simulink model "psk_model_coded"  (R2023a)
settings: Solver=FixedStepDiscrete  StartTime=0.0  StopTime=1e5  FixedStep=1  RelTol=1e-3
values from neighbouring files (symbols this model uses):
  M = M_values(mod_idx)    [run_ber_sweep.m]
undefined symbols (not defined in the file or in its folder): dvbs2ldpc, Ts
libraries: commsink2 x2, simulink x2, commblkcod2 x2, commcnvcod2 x2, commdigbbndpm3 x2, commchan3 x1, commrandsrc3 x1
settings Model: Creator=aleks  LastModifiedBy=aleks

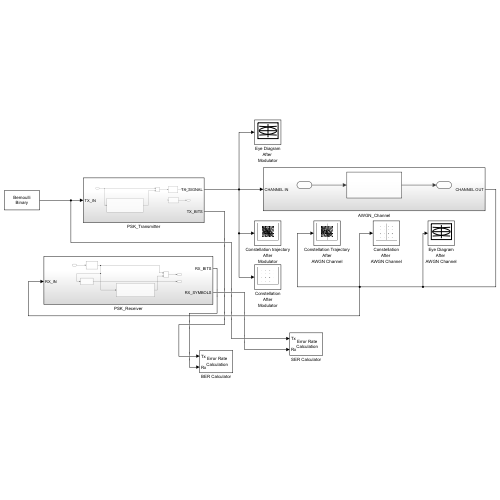
[thumbnail: Simulink's stored preview of the top-level diagram]
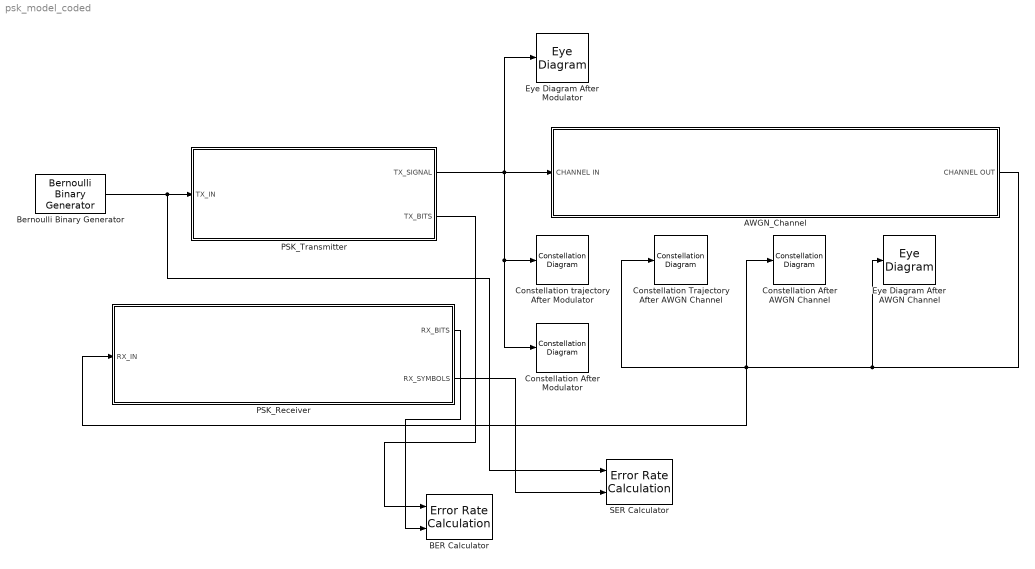
== system psk_model_coded ==
  AWGN_Channel : Subsystem
  BER Calculator : commsink2/Error Rate Calculation  N=0  st_delay=0  cp_mode=Entire frame  subframe=[]  PMode=Workspace  WsName=ber_out  RsMode2=off  stop=off  numErr=100  maxBits=1e6
  Bernoulli Binary Generator : commrandsrc3/Bernoulli Binary Generator  ProbabilityOfZero=bern_prob  SeedSource=Auto  Seed=0  SampleTime=Ts  SamplesPerFrame=1  OutputDataType=double  SimulateUsing=Interpreted execution
  Constellation After Modulator : ConstellationDiagram  WindowPosition=[2.000000,50.000000,766.000000,881.000000,]  Visible=on  ScopeFrameLocation=window  SymbolsToDisplaySource=Property  SymbolsToDisplay=1000  XLimits=[-1.46,1.46]  YLimits=[-1.38,1.38]  ShowReferenceConstellation=off
  Constellation After AWGN Channel : ConstellationDiagram  WindowPosition=[770.000000,50.000000,766.000000,881.000000,]  Visible=on  ScopeFrameLocation=window  SymbolsToDisplaySource=Property  SymbolsToDisplay=1000  XLimits=[-1.46,1.46]  YLimits=[-1.38,1.38]  ShowReferenceConstellation=off
  Constellation Trajectory After AWGN Channel : ConstellationDiagram  WindowPosition=[770.000000,50.000000,766.000000,881.000000,]  Visible=on  ScopeFrameLocation=window  SymbolsToDisplaySource=Property  SymbolsToDisplay=1000  ReferenceConstellation=QPSK  XLimits=[-1.46,1.46]  YLimits=[-1.38,1.38]  ShowTrajectory=on  ShowReferenceConstellation=off
  Constellation trajectory After Modulator : ConstellationDiagram  WindowPosition=[2.000000,50.000000,766.000000,881.000000,]  Visible=on  ScopeFrameLocation=window  SymbolsToDisplaySource=Property  SymbolsToDisplay=1000  ReferenceConstellation=QPSK  XLimits=[-1.46,1.46]  YLimits=[-1.38,1.38]  ShowTrajectory=on  ShowReferenceConstellation=off
  Eye Diagram After AWGN Channel : EyeDiagram
  Eye Diagram After Modulator : EyeDiagram
  PSK_Receiver : Subsystem
  PSK_Transmitter : Subsystem
  SER Calculator : commsink2/Error Rate Calculation  N=0  st_delay=0  cp_mode=Entire frame  subframe=[]  PMode=Workspace  WsName=ser_out  RsMode2=off  stop=off  numErr=100  maxBits=1e6
  wires:
  PSK_Transmitter/1(TX_SIGNAL) -> Constellation After Modulator/1, Constellation trajectory After Modulator/1, Eye Diagram After Modulator/1, AWGN_Channel/1(CHANNEL IN)
  AWGN_Channel/1(CHANNEL OUT) -> Eye Diagram After AWGN Channel/1, PSK_Receiver/1(RX_IN), Constellation After AWGN Channel/1, Constellation Trajectory After AWGN Channel/1
  Bernoulli Binary Generator/1 -> SER Calculator/1, PSK_Transmitter/1(TX_IN)
  PSK_Receiver/1(RX_BITS) -> BER Calculator/2
  PSK_Transmitter/2(TX_BITS) -> BER Calculator/1
  PSK_Receiver/2(RX_SYMBOLS) -> SER Calculator/2

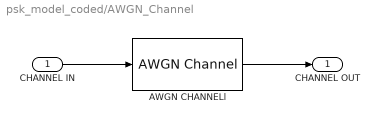
== system psk_model_coded/AWGN_Channel ==
  CHANNEL IN : Inport
  AWGN CHANNELl : commchan3/AWGN Channel  LegacyMode=off  NoiseMethod="Signal to noise ratio  (Eb/No)"  noiseMode="Signal to noise ratio  (SNR)"  EbNo=EbNo_curr  EsNo=10  SNR=10  BitsPerSymbol=log2(M)  SignalPower=1  SamplesPerSymbol=1  SymbolPeriod=1  VarianceSource=Parameter  Variance=1  RandomStream=Global stream  Seed=67  SimulateUsing=Code generation
  CHANNEL OUT : Outport
  wires:
  CHANNEL IN/1 -> AWGN CHANNELl/1
  AWGN CHANNELl/1 -> CHANNEL OUT/1

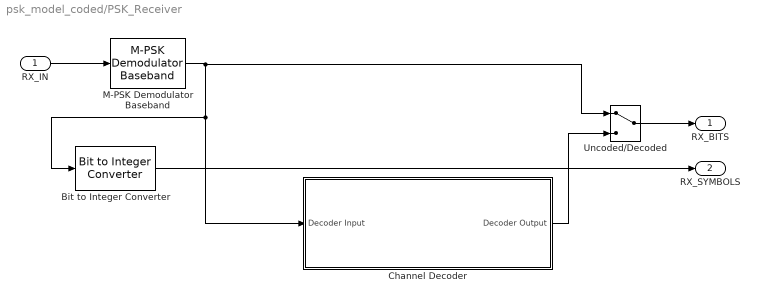
== system psk_model_coded/PSK_Receiver ==
  RX_IN : Inport
  Bit to Integer Converter : simulink/Logic and Bit Operations/Bit to Integer Converter  nbits=log2(M)  bitOrder=MSB first  signedOutputValues=Unsigned  outDtype=Inherit via internal rule  outDtypeSigned=Inherit via internal rule
  Channel Decoder : Subsystem
  M-PSK Demodulator Baseband : commdigbbndpm3/M-PSK Demodulator Baseband  M=M  OutType=Bit  DecType=Hard decision  VarSource=Dialog  Variance=1  Dec=Gray  Mapping=[0:7]  Ph=phase_offset  outDtype1=Inherit via internal rule  outDtype2=Inherit via internal rule  derotateFactorWordLen=16  derotateFactorDataTypeStr=Inherit: Same word length as input  derotateFactorLastDataTypeStr=Inherit: Same word length as input
  Uncoded/Decoded : ManualSwitch
  RX_BITS : Outport
  RX_SYMBOLS : Outport  Port=2
  wires:
  RX_IN/1 -> M-PSK Demodulator Baseband/1
  Bit to Integer Converter/1 -> RX_SYMBOLS/1
  M-PSK Demodulator Baseband/1 -> Uncoded/Decoded/1, Channel Decoder/1(Decoder Input), Bit to Integer Converter/1
  Channel Decoder/1(Decoder Output) -> Uncoded/Decoded/2
  Uncoded/Decoded/1 -> RX_BITS/1

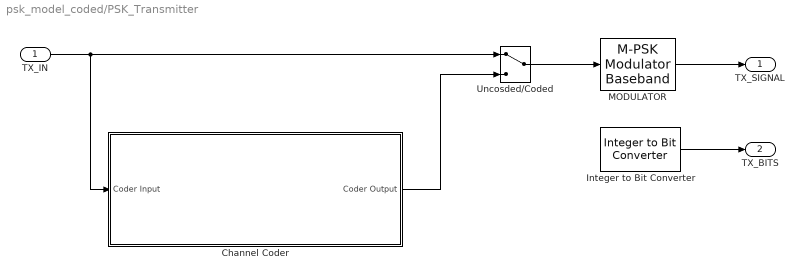
== system psk_model_coded/PSK_Transmitter ==
  TX_IN : Inport
  Channel Coder : Subsystem
  Integer to Bit Converter : simulink/Logic and Bit Operations/Integer to Bit Converter  nbits=log2(M)  signedInputValues=Unsigned  bitOrder=MSB first  outDtype=Inherit via internal rule
  MODULATOR : commdigbbndpm3/M-PSK Modulator Baseband  M=M  InType=Integer  Enc=Gray  Mapping=[0:7]  Ph=phase_offset  outDtype=double  outWordLen=16  outUDDataType=sfix(16)  outFracLenMode=Best precision  outFracLen=15  outDataTypeStr=double  outLastDataTypeStr=double
  Uncosded/Coded : ManualSwitch
  TX_SIGNAL : Outport
  TX_BITS : Outport  Port=2
  wires:
  MODULATOR/1 -> TX_SIGNAL/1
  Integer to Bit Converter/1 -> TX_BITS/1
  TX_IN/1 -> Channel Coder/1(Coder Input), Uncosded/Coded/1
  Channel Coder/1(Coder Output) -> Uncosded/Coded/2
  Uncosded/Coded/1 -> MODULATOR/1

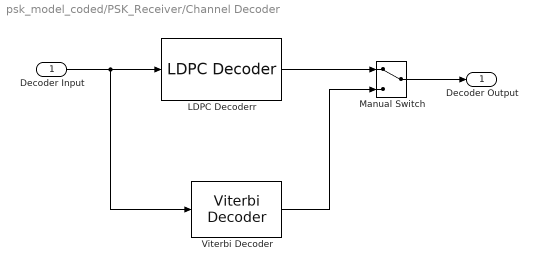
== system psk_model_coded/PSK_Receiver/Channel Decoder ==
  Decoder Input : Inport
  LDPC Decoderr : commblkcod2/LDPC Decoder  ParityCheckMat=dvbs2ldpc(1/2)  OutputFmt=Information part  DecisionType=Hard decision  OutputDataType=double  NumIter=50  DoParityCheck=off  OutputNumIter=off  OutputFinalChecks=off
  Manual Switch : ManualSwitch
  Viterbi Decoder : commcnvcod2/Viterbi Decoder  trellis=poly2trellis(7, [171 133])  isPunctured=off  punctureVector=[1; 1; 0; 1; 0; 1]  erasures=off  dectype=Hard decision  nsdecb=4  runSigValErrCheck=off  tbdepth=34  opmode=Continuous  reset=off  delayedResetAction=off  smWordLength=16  outDataType=Inherit via internal rule
  Decoder Output : Outport
  wires:
  Decoder Input/1 -> Viterbi Decoder/1, LDPC Decoderr/1
  LDPC Decoderr/1 -> Manual Switch/1
  Viterbi Decoder/1 -> Manual Switch/2
  Manual Switch/1 -> Decoder Output/1

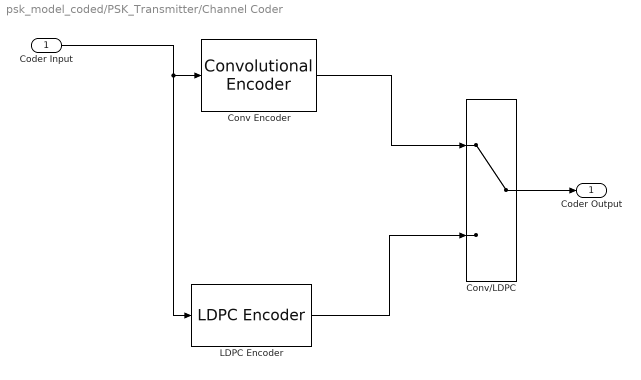
== system psk_model_coded/PSK_Transmitter/Channel Coder ==
  Coder Input : Inport
  Conv Encoder : commcnvcod2/Convolutional Encoder  trellis=poly2trellis(7, [171 133])  opMode=Continuous  DelayedResetAction=off  hasIniStPort=off  hasFinStPort=off  usePuncVector=off  punctureVector=[1; 1; 0; 1; 0; 1]  reset=Unused parameter value
  Conv/LDPC : ManualSwitch
  LDPC Encoder : commblkcod2/LDPC Encoder  ParityCheckMat=dvbs2ldpc(1/2)
  Coder Output : Outport
  wires:
  Conv Encoder/1 -> Conv/LDPC/1
  LDPC Encoder/1 -> Conv/LDPC/2
  Coder Input/1 -> LDPC Encoder/1, Conv Encoder/1
  Conv/LDPC/1 -> Coder Output/1
